simulink model "sampleModel163"  (R2021b)
settings: Solver=VariableStepAuto  StartTime=0.0  StopTime=10.0  RelTol=1e-3
undefined symbols (not defined in the file or in its folder): DiscIntNeverNeededParam
libraries: simulink x8, slpidlib x1
settings Model: Creator=user  LastModifiedBy=user

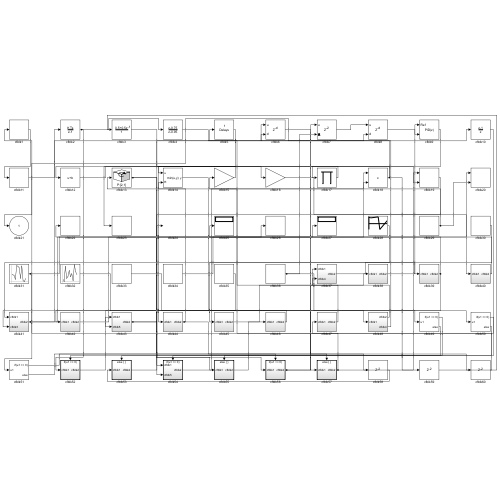
[thumbnail: Simulink's stored preview of the top-level diagram]
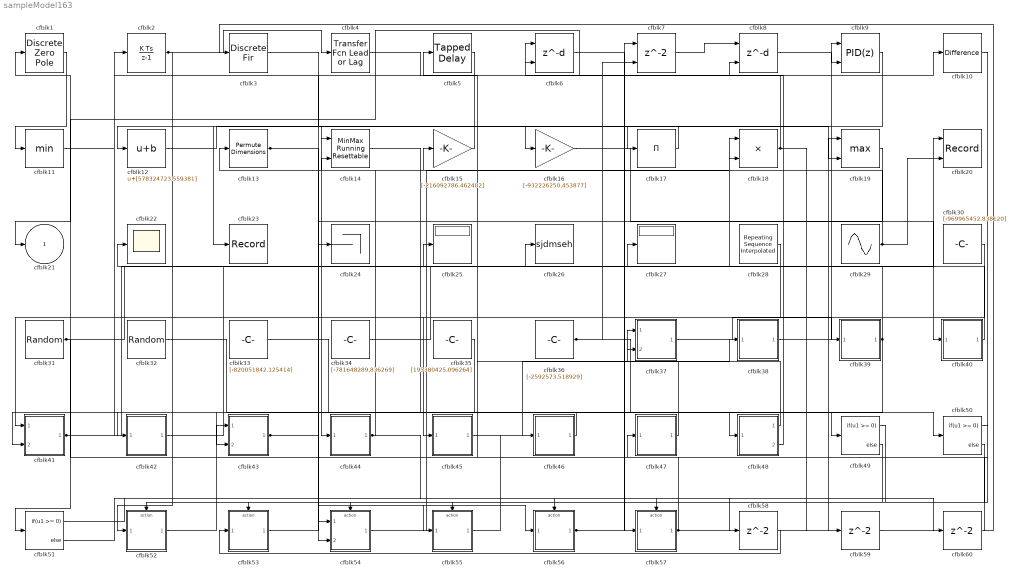
== system sampleModel163 ==
  cfblk1 : DiscreteZeroPole  Poles=[0 0.5]  Gain=1
  cfblk10 : simulink/Discrete/Difference  ICPrevInput=0.0  OutMin=[]  OutMax=[]  OutDataTypeStr=Inherit: Inherit via back propagation  OutDataType=fixdt(1, 16)  OutScaling=2^-10  DoSatur=off
  cfblk11 : MinMax
  cfblk12 : Bias  Bias=[578324723.559381]
  cfblk13 : PermuteDimensions
  cfblk14 : simulink/Math Operations/MinMax Running Resettable  Function=min  vinit=0.0
  cfblk15 : Gain  Gain=[-216092786.462482]
  cfblk16 : Gain  Gain=[-932226250.453877]
  cfblk17 : Product  Inputs=*
  cfblk18 : Product  Inputs=**
  cfblk19 : MinMax  Function=max  Inputs=2
  cfblk2 : DiscreteIntegrator  ICPrevOutput=DiscIntNeverNeededParam  ICPrevScaledInput=DiscIntNeverNeededParam
  cfblk20 : Record  FileSettingsInternal="{\"entries\":[{\"content\":{\"excelSettings\":{\"content\":{},\"type\":\"Streamout.ExcelSettings\"}},\"type\":\"Streamout.FileSettingStorage\",\"uuid\":\"06ed781e-12cb-4e05-8bb1-7b1aca927446\"}],\"packageUris\":[\"http://schema.mathworks.com/mf0/streamout_blocks/R2020a\"],\"version\":\"1.0\"}"  Layout=[1 1]  SignalsInternal="{\"entries\":[{\"content\":{\"signals\":[{\"content\":{\"blockPath\":[\"sampleModel163/cfblk20\"],\"channel\":[],\"dimensions\":[1],\"domain\":\"sampleModel163/cfblk20\",\"lineColor\":\"#a2142f\",\"plots\":[1],\"port\":1,\"sid\":[\"\"],\"signalID\":6164,\"signalName\":\"cfblk31\"},\"type\":\"RecordBlkView.Signal\",\"uuid\":\"f8e4e534-be1f-4f40-ab34-d8d78202847f\"},{\"content\":{\"blockPath\":[\"sampleModel163/cfblk20\"],\"channel\":[],\"dimensions\":[1],\"domain\":\"sampleModel163/cfblk20\",\"lineColor\":\"#139fff\",\"plots\":[1],\"port\":2,\"sid\":[\"\"],\"signalID\":6168,\"signalName\":\"cfblk29\"},\"type\":\"RecordBlkView.Signal\",\"uuid\":\"e7af1ba5-8239-4218-b823-7982c55ee47a\"}]},\"type\":\"RecordBlkView.InputSignals\",\"uuid\":\"71169161-2672-4fe2-b37d-7ccbea77738d\"}],\"packageUris\":[\"http://schema.mathworks.com/mf0/streamout_blocks/R2020a\"],\"version\":\"1.0\"}"  VisualizationBindings="{\"xyplotplugin\":{\"info\":[{\"series\":[{\"bindingParametersList\":[{\"parameter\":\"X-Axis\",\"signalID\":6164,\"signalName\":\"cfblk31\"},{\"parameter\":\"Y-Axis\",\"signalID\":6168,\"signalName\":\"cfblk29\"}],\"seriesID\":65213}],\"subplotID\":1}]}}"  CompatibilityTag=XY
  cfblk22 : Scope
  cfblk23 : Record  FileSettingsInternal="{\"entries\":[{\"content\":{\"excelSettings\":{\"content\":{},\"type\":\"Streamout.ExcelSettings\"}},\"type\":\"Streamout.FileSettingStorage\",\"uuid\":\"58f81f9b-3091-4bfb-8b59-2bbb88b916ca\"}],\"packageUris\":[\"http://schema.mathworks.com/mf0/streamout_blocks/R2020a\"],\"version\":\"1.0\"}"  SignalsInternal="{\"entries\":[{\"content\":{\"signals\":[{\"content\":{\"blockPath\":[\"sampleModel163/cfblk23\"],\"channel\":[],\"dimensions\":[1],\"domain\":\"sampleModel163/cfblk23\",\"lineColor\":\"#77ac30\",\"plots\":[1],\"port\":1,\"sid\":[\"\"],\"signalID\":6172,\"signalName\":\"cfblk15\"},\"type\":\"RecordBlkView.Signal\",\"uuid\":\"70741671-3e54-430a-8378-0fd8a2290cdd\"}]},\"type\":\"RecordBlkView.InputSignals\",\"uuid\":\"9b4d039f-f325-4278-9c4c-6e897f4be92f\"}],\"packageUris\":[\"http://schema.mathworks.com/mf0/streamout_blocks/R2020a\"],\"version\":\"1.0\"}"  VisualizationBindings="{\"sparklinesplugin\":{\"info\":[{\"bindingParametersList\":[],\"subplotID\":1}]}}"
  cfblk24 : Terminator
  cfblk25 : Display
  cfblk26 : ToWorkspace  VariableName=sjdmseh  SaveFormat=Timeseries  SampleTime=-1
  cfblk27 : Display
  cfblk28 : simulink/Sources/Repeating Sequence Interpolated  OutValues=[732237862.011595, 651862154.247679, 790634428.736061, -683577419.682949, 318530524.873353]  TimeValues=[0 0.1 0.5 0.6 1].'  LookUpMeth=Use Input Nearest  tsamp=0.01  OutMin=[]  OutMax=[]  OutDataTypeStr=double  OutputDataTypeScalingMode=double  OutDataType=fixdt(0,8)  OutScaling=2^-10
  cfblk29 : Sin  Amplitude=[237996314.425898]  Bias=[21398783.004836]  SampleTime=0
  cfblk3 : DiscreteFir  SampleTime=1
  cfblk30 : Constant  Value=[-969965452.838120]  SampleTime=1
  cfblk31 : RandomNumber  Mean=[-19567.481043]  Variance=[38445.475397]  Seed=[599770509.000000]  SampleTime=0.1
  cfblk32 : UniformRandomNumber  Minimum=[-4062021500.164922]  Maximum=[206796190.518302]  Seed=[57462466.000000]  SampleTime=0.1
  cfblk33 : Constant  Value=[-820051842.125414]  SampleTime=1
  cfblk34 : Constant  Value=[-781648289.836269]  SampleTime=1
  cfblk35 : Constant  Value=[195380425.096264]  SampleTime=1
  cfblk36 : Constant  Value=[-2592573.518929]  SampleTime=1
  cfblk37 : Subsystem
  cfblk38 : Subsystem
  cfblk39 : Subsystem
  cfblk4 : simulink/Discrete/Transfer Fcn Lead or Lag  PoleZ=0.95  ZeroZ=0.75  ICPrevOutput=0.0  ICPrevInput=0.0  DoSatur=off
      settings: SourceProductBaseCode=SL
  cfblk40 : Subsystem
  cfblk41 : Subsystem
  cfblk42 : Subsystem
  cfblk43 : Subsystem
  cfblk44 : Subsystem
  cfblk45 : Subsystem
  cfblk46 : Subsystem
  cfblk47 : Subsystem
  cfblk48 : Subsystem
  cfblk49 : If  IfExpression=u1 >= 0  SampleTime=1
  cfblk5 : simulink/Discrete/Tapped Delay  vinit=0.0  samptime=-1  NumDelays=1  DelayOrder=Oldest  includeCurrent=off
  cfblk50 : If  IfExpression=u1 >= 0  SampleTime=1
  cfblk51 : If  IfExpression=u1 >= 0  SampleTime=1
  cfblk52 : Subsystem  TreatAsAtomicUnit=on
  cfblk53 : Subsystem  TreatAsAtomicUnit=on
  cfblk54 : Subsystem  TreatAsAtomicUnit=on
  cfblk55 : Subsystem  TreatAsAtomicUnit=on
  cfblk56 : Subsystem  TreatAsAtomicUnit=on
  cfblk57 : Subsystem  TreatAsAtomicUnit=on
  cfblk58 : Delay  SampleTime=1
  cfblk59 : Delay  SampleTime=1
  cfblk6 : Delay  DelayLengthSource=Input port  SampleTime=1
      settings: InputPortMap=u0,p1
  cfblk60 : Delay  SampleTime=1
  cfblk7 : Delay  ShowEnablePort=on  SampleTime=1
      settings: InputPortMap=u0,e6
  cfblk8 : Delay  DelayLengthSource=Input port  SampleTime=1
      settings: InputPortMap=u0,p1
  cfblk9 : slpidlib/PID Controller (2DOF)  Controller=PID  Form=Parallel  TimeDomain=Discrete-time  UseExternalTs=off  SampleTime=1  IntegratorMethod=Forward Euler  FilterMethod=Forward Euler  ControllerParametersSource=internal  P=1  I=1  D=0  UseFilter=on  N=100  b=1  c=1  TunerSelectOption=Transfer Function Based (PID Tuner App)  InitialConditionSource=internal  InitialConditionForIntegrator=0  InitialConditionForFilter=0  DifferentiatorICPrevScaledInput=0  ExternalReset=none  TrackingMode=off  Kt=1  LimitOutput=off  SatLimitsSource=internal  UpperSaturationLimit=inf  LowerSaturationLimit=-inf  LinearizeAsGain=off  AntiWindupMode=none  Kb=1  POutMin=[]  POutMax=[]  IOutMin=[]  IOutMax=[]  DOutMin=[]  DOutMax=[]  NOutMin=[]  NOutMax=[]  bOutMin=[]  bOutMax=[]  cOutMin=[]  cOutMax=[]  SumOutMin=[]  SumOutMax=[]  SaturationOutMin=[]  SaturationOutMax=[]  PParamMin=[]  PParamMax=[]  IParamMin=[]  IParamMax=[]  DParamMin=[]  DParamMax=[]  NParamMin=[]  NParamMax=[]  bParamMin=[]  bParamMax=[]  cParamMin=[]  cParamMax=[]  KbParamMin=[]  KbParamMax=[]  KtParamMin=[]  KtParamMax=[]  KbOutMin=[]  KbOutMax=[]  KtOutMin=[]  KtOutMax=[]  IntegratorOutMin=[]  IntegratorOutMax=[]  FilterOutMin=[]  FilterOutMax=[]  SumI1OutMin=[]  SumI1OutMax=[]  SumI2OutMin=[]  SumI2OutMax=[]  SumI3OutMin=[]  SumI3OutMax=[]  SumI4OutMin=[]  SumI4OutMax=[]  SumDOutMin=[]  SumDOutMax=[]  Sum1OutMin=[]  Sum1OutMax=[]  Sum2OutMin=[]  Sum2OutMax=[]  Sum3OutMin=[]  Sum3OutMax=[]  DifferentiatorOutMin=[]  DifferentiatorOutMax=[]  FilterDiffOutCoefMin=[]  FilterDiffOutCoefMax=[]  ReciprocalOutMin=[]  ReciprocalOutMax=[]  SumDenOutMin=[]  SumDenOutMax=[]  SumNumOutMin=[]  SumNumOutMax=[]  DivideOutMin=[]  DivideOutMax=[]  UdiffTsProdOutMin=[]  UdiffTsProdOutMax=[]  NTsProdOutMin=[]  NTsProdOutMax=[]  UintegralTsProdOutMin=[]  UintegralTsProdOutMax=[]  UngainTsProdOutMin=[]  UngainTsProdOutMax=[]  IntegratorContinuousStateAttributes=''  IntegratorStateMustResolveToSignalObject=off  IntegratorRTWStateStorageClass=Auto  FilterContinuousStateAttributes=''  FilterStateMustResolveToSignalObject=off  FilterRTWStateStorageClass=Auto  ParallelPVariant=InternalParameters  IdealPVariant=Disabled  IVariant=InternalParameters  DVariant=InternalParameters  bVariant=InternalParameters  cVariant=InternalParameters  IntegratorVariant=Discrete  SatVariant=Disabled  AWVariant=Passthrough  PCopyVariant=Disabled  TRVariant=Disabled  FdbkBlocksVariant=Forward  IdealPFdbkVariant=Disabled  SatFdbkVariant=Disabled  DerivativeFilterVariant=ForwardEulerFilter  NVariant=InternalParameters  NCopyVariant=Disabled  FilterICVariant=InternalICsFilter  IntegratorICVariant=InternalICs  ExternalResetVariant=Disabled  TRSumVariant=Passthrough  SumFdbkVariant=Disabled  SumVariant=Sum_PID  TsampFilterVariant=InternalTs  TsampNgainVariant=Passthrough  TsampIntegralVariant=Passthrough  ExternalSaturationOutDataTypeStr=Inherit: Same as second input
      settings: SourceProductBaseCode=SL
  cfblk21 : Outport
  wires:
  cfblk29/1 -> cfblk13/1, cfblk20/2
  cfblk30/1 -> cfblk41/1(cfblk1)
  cfblk38/1(cfblk2) -> cfblk9/1
  cfblk15/1 -> cfblk23/1
  cfblk5/1 -> cfblk44/1(cfblk1)
  cfblk8/1 -> cfblk9/2
  cfblk34/1 -> cfblk26/1
  cfblk36/1 -> cfblk50/1, cfblk7/2
  cfblk1/1 -> cfblk11/1
  cfblk41/1(cfblk2) -> cfblk27/1, cfblk10/1
  cfblk40/1(cfblk2) -> cfblk22/1
  cfblk35/1 -> cfblk41/2(cfblk3)
  cfblk37/1(cfblk2) -> cfblk39/1(cfblk1)
  cfblk32/1 -> cfblk49/1
  cfblk46/1(cfblk2) -> cfblk42/1(cfblk1)
  cfblk2/1 -> cfblk4/1, cfblk52/1(cfblk1)
  cfblk18/1 -> cfblk21/1, cfblk14/1, cfblk59/1
  cfblk31/1 -> cfblk20/1, cfblk51/1
  cfblk54/1(cfblk2) -> cfblk18/1
  cfblk55/1(cfblk2) -> cfblk46/1(cfblk1)
  cfblk39/1(cfblk2) -> cfblk25/1, cfblk43/2(cfblk5)
  cfblk48/1(cfblk2) -> cfblk15/1
  cfblk10/1 -> cfblk47/1(cfblk1)
  cfblk44/1(cfblk2) -> cfblk14/2, cfblk60/1
  cfblk28/1 -> cfblk45/1(cfblk1)
  cfblk42/1(cfblk2) -> cfblk18/2
  cfblk16/1 -> cfblk40/1(cfblk1)
  cfblk57/1(cfblk2) -> cfblk19/1, cfblk1/1
  cfblk45/1(cfblk2) -> cfblk37/1(cfblk1)
  cfblk14/1 -> cfblk48/1(cfblk1)
  cfblk9/1 -> cfblk17/1
  cfblk52/1(cfblk2) -> cfblk43/1(cfblk1)
  cfblk53/1(cfblk2) -> cfblk24/1
  cfblk17/1 -> cfblk12/1
  cfblk43/1(cfblk2) -> cfblk6/1, cfblk56/1(cfblk1)
  cfblk7/1 -> cfblk8/1
  cfblk12/1 -> cfblk16/1
  cfblk56/1(cfblk2) -> cfblk7/1, cfblk38/1(cfblk1)
  cfblk13/1 -> cfblk54/1(cfblk1), cfblk55/1(cfblk1)
  cfblk3/1 -> cfblk19/2
  cfblk4/1 -> cfblk8/2
  cfblk19/1 -> cfblk54/2(cfblk5)
  cfblk47/1(cfblk2) -> cfblk37/2(cfblk4)
  cfblk33/1 -> cfblk57/1(cfblk1)
  cfblk11/1 -> cfblk2/1
  cfblk48/2(cfblk4) -> cfblk6/2
  cfblk49/1 -> cfblk52/Action
  cfblk49/2 -> cfblk53/Action
  cfblk50/1 -> cfblk54/Action
  cfblk50/2 -> cfblk55/Action
  cfblk51/1 -> cfblk56/Action
  cfblk51/2 -> cfblk57/Action
  cfblk6/1 -> cfblk58/1
  cfblk58/1 -> cfblk53/1(cfblk1)
  cfblk59/1 -> cfblk3/1
  cfblk60/1 -> cfblk5/1

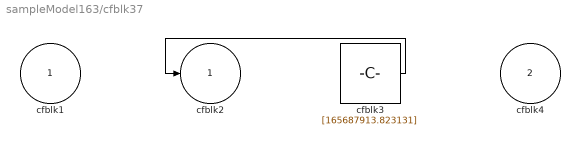
== system sampleModel163/cfblk37 ==
  cfblk1 : Inport
  cfblk4 : Inport  Port=2
  cfblk3 : Constant  Value=[165687913.823131]  SampleTime=1
  cfblk2 : Outport
  wires:
  cfblk3/1 -> cfblk2/1

== system sampleModel163/cfblk38 ==
  cfblk1 : Inport
  cfblk3 : Math  Operator=10^u  SaturateOnIntegerOverflow=on
  cfblk2 : Outport
  wires:
  cfblk1/1 -> cfblk3/1
  cfblk3/1 -> cfblk2/1

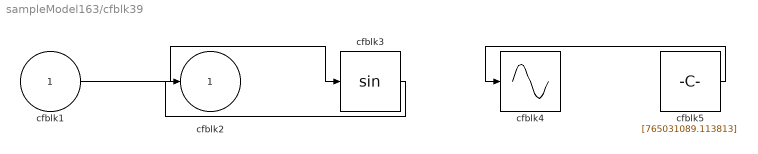
== system sampleModel163/cfblk39 ==
  cfblk1 : Inport
  cfblk3 : Trigonometry
  cfblk4 : Sin  TimeSource=Use external signal  SampleTime=0
  cfblk5 : Constant  Value=[765031089.113813]  SampleTime=1
  cfblk2 : Outport
  wires:
  cfblk1/1 -> cfblk3/1
  cfblk3/1 -> cfblk2/1
  cfblk5/1 -> cfblk4/1

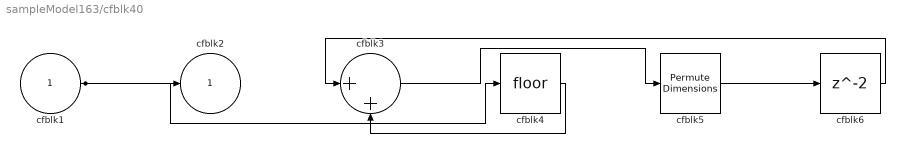
== system sampleModel163/cfblk40 ==
  cfblk1 : Inport
  cfblk3 : Sum  Inputs=|++
  cfblk4 : Rounding
  cfblk5 : PermuteDimensions
  cfblk6 : Delay  SampleTime=1
  cfblk2 : Outport
  wires:
  cfblk1/1 -> cfblk4/1, cfblk2/1
  cfblk4/1 -> cfblk3/2
  cfblk3/1 -> cfblk5/1
  cfblk5/1 -> cfblk6/1
  cfblk6/1 -> cfblk3/1

== system sampleModel163/cfblk41 ==
  cfblk1 : Inport
  cfblk3 : Inport  Port=2
  cfblk2 : Outport
  wires:
  cfblk1/1 -> cfblk2/1

== system sampleModel163/cfblk42 ==
  cfblk1 : Inport
  cfblk3 : Sum  Inputs=+
  cfblk2 : Outport
  wires:
  cfblk3/1 -> cfblk2/1
  cfblk1/1 -> cfblk3/1

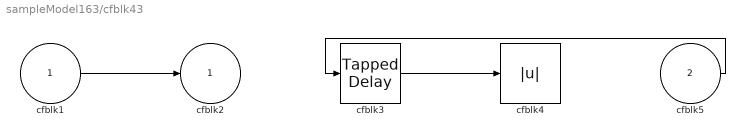
== system sampleModel163/cfblk43 ==
  cfblk1 : Inport
  cfblk5 : Inport  Port=2
  cfblk3 : simulink/Discrete/Tapped Delay  vinit=0.0  samptime=-1  NumDelays=1  DelayOrder=Oldest  includeCurrent=off
  cfblk4 : Abs
  cfblk2 : Outport
  wires:
  cfblk5/1 -> cfblk3/1
  cfblk3/1 -> cfblk4/1
  cfblk1/1 -> cfblk2/1

== system sampleModel163/cfblk44 ==
  cfblk1 : Inport
  cfblk3 : ComplexToMagnitudeAngle
  cfblk2 : Outport
  wires:
  cfblk1/1 -> cfblk3/1
  cfblk3/1 -> cfblk2/1

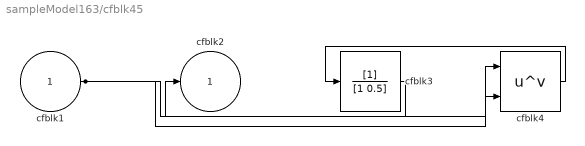
== system sampleModel163/cfblk45 ==
  cfblk1 : Inport
  cfblk3 : DiscreteFilter  SampleTime=1
  cfblk4 : Math  Operator=pow  SaturateOnIntegerOverflow=on
  cfblk2 : Outport
  wires:
  cfblk4/1 -> cfblk3/1
  cfblk3/1 -> cfblk2/1
  cfblk1/1 -> cfblk4/1, cfblk4/2

== system sampleModel163/cfblk46 ==
  cfblk1 : Inport
  cfblk3 : Delay  DelayLengthSource=Input port  SampleTime=1
      settings: InputPortMap=u0,p1
  cfblk2 : Outport
  wires:
  cfblk1/1 -> cfblk3/1, cfblk3/2
  cfblk3/1 -> cfblk2/1

== system sampleModel163/cfblk47 ==
  cfblk1 : Inport
  cfblk3 : ComplexToMagnitudeAngle
  cfblk2 : Outport
  wires:
  cfblk1/1 -> cfblk3/1
  cfblk3/1 -> cfblk2/1

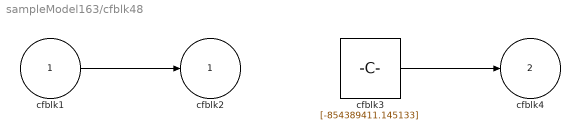
== system sampleModel163/cfblk48 ==
  cfblk1 : Inport
  cfblk3 : Constant  Value=[-854389411.145133]  SampleTime=1
  cfblk2 : Outport
  cfblk4 : Outport  Port=2
  wires:
  cfblk3/1 -> cfblk4/1
  cfblk1/1 -> cfblk2/1

== system sampleModel163/cfblk52 ==
  cfblk1 : Inport
  Action Port : ActionPort  ActionPortLabel=if(u1 >= 0)
  cfblk3 : Constant  Value=[-885075560.792132]  SampleTime=1
  cfblk2 : Outport
  wires:
  cfblk1/1 -> cfblk2/1

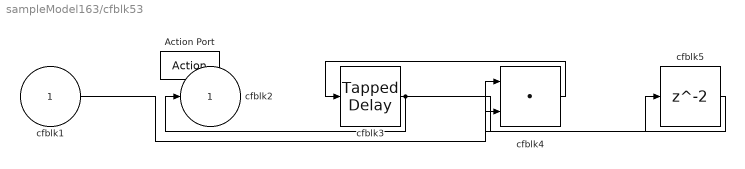
== system sampleModel163/cfblk53 ==
  cfblk1 : Inport
  Action Port : ActionPort  ActionPortLabel=else
  cfblk3 : simulink/Discrete/Tapped Delay  vinit=0.0  samptime=-1  NumDelays=1  DelayOrder=Oldest  includeCurrent=off
  cfblk4 : DotProduct  InputSameDT=on  OutDataTypeStr=Inherit: Inherit via internal rule
  cfblk5 : Delay
  cfblk2 : Outport
  wires:
  cfblk4/1 -> cfblk3/1
  cfblk3/1 -> cfblk2/1, cfblk5/1
  cfblk1/1 -> cfblk4/1
  cfblk5/1 -> cfblk4/2

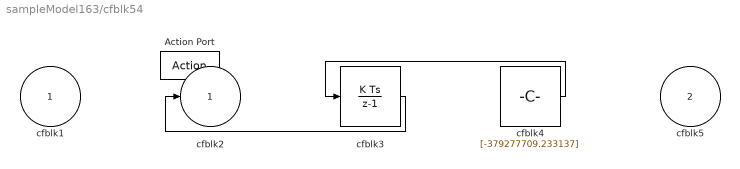
== system sampleModel163/cfblk54 ==
  cfblk1 : Inport
  cfblk5 : Inport  Port=2
  Action Port : ActionPort  ActionPortLabel=if(u1 >= 0)
  cfblk3 : DiscreteIntegrator  SampleTime=-1  ICPrevOutput=DiscIntNeverNeededParam  ICPrevScaledInput=DiscIntNeverNeededParam
  cfblk4 : Constant  Value=[-379277709.233137]  SampleTime=1
  cfblk2 : Outport
  wires:
  cfblk3/1 -> cfblk2/1
  cfblk4/1 -> cfblk3/1

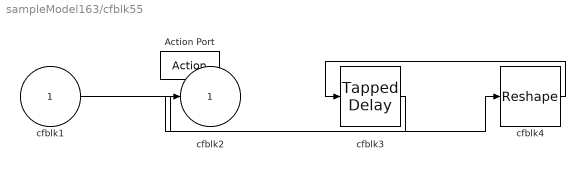
== system sampleModel163/cfblk55 ==
  cfblk1 : Inport
  Action Port : ActionPort  ActionPortLabel=else
  cfblk3 : simulink/Discrete/Tapped Delay  vinit=0.0  samptime=-1  NumDelays=1  DelayOrder=Oldest  includeCurrent=off
  cfblk4 : Reshape
  cfblk2 : Outport
  wires:
  cfblk4/1 -> cfblk3/1
  cfblk1/1 -> cfblk4/1
  cfblk3/1 -> cfblk2/1

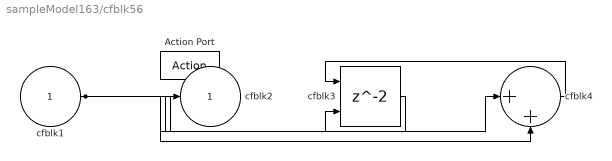
== system sampleModel163/cfblk56 ==
  cfblk1 : Inport
  Action Port : ActionPort  ActionPortLabel=if(u1 >= 0)
  cfblk3 : Delay  ShowEnablePort=on
      settings: InputPortMap=u0,e6
  cfblk4 : Sum  Inputs=|++
  cfblk2 : Outport
  wires:
  cfblk1/1 -> cfblk4/1, cfblk3/2, cfblk4/2
  cfblk4/1 -> cfblk3/1
  cfblk3/1 -> cfblk2/1

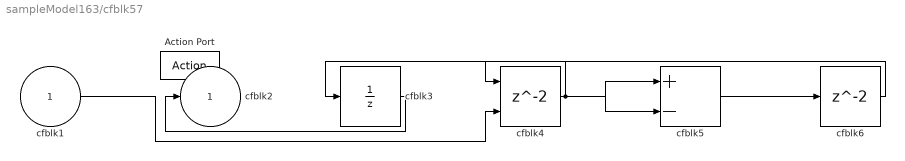
== system sampleModel163/cfblk57 ==
  cfblk1 : Inport
  Action Port : ActionPort  ActionPortLabel=else
  cfblk3 : UnitDelay  SampleTime=-1  HasFrameUpgradeWarning=on
  cfblk4 : Delay  ShowEnablePort=on
      settings: InputPortMap=u0,e6
  cfblk5 : Sum  Inputs=+-
  cfblk6 : Delay
  cfblk2 : Outport
  wires:
  cfblk3/1 -> cfblk2/1
  cfblk1/1 -> cfblk4/2
  cfblk4/1 -> cfblk5/1, cfblk3/1, cfblk5/2
  cfblk5/1 -> cfblk6/1
  cfblk6/1 -> cfblk4/1
